simulink model "Vereinfachte_Drehtellersteuerung"  (R2021b)
settings: Solver=ode3  StartTime=0.0  StopTime=10.0  FixedStep=0.01  RelTol=1e-3
values from neighbouring files (symbols this model uses):
  A = 5    [Parametriesierung.m]
  I = 0.5    [Parametriesierung.m]
  igetr = 1080    [Parametriesierung.m]
  K = 8    [Parametriesierung.m]
  MRK = 1    [Parametriesierung.m]
  PHI = 0.001    [Parametriesierung.m]
  Ra = 40    [Parametriesierung.m]
  U = 24    [Parametriesierung.m]
settings Model: Creator=mwjae  LastModifiedBy=mwjae

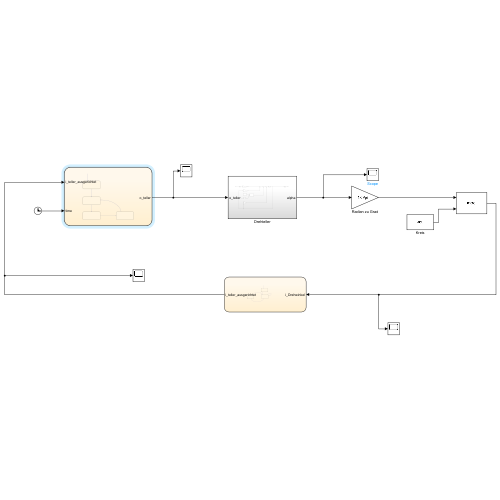
[thumbnail: Simulink's stored preview of the top-level diagram]
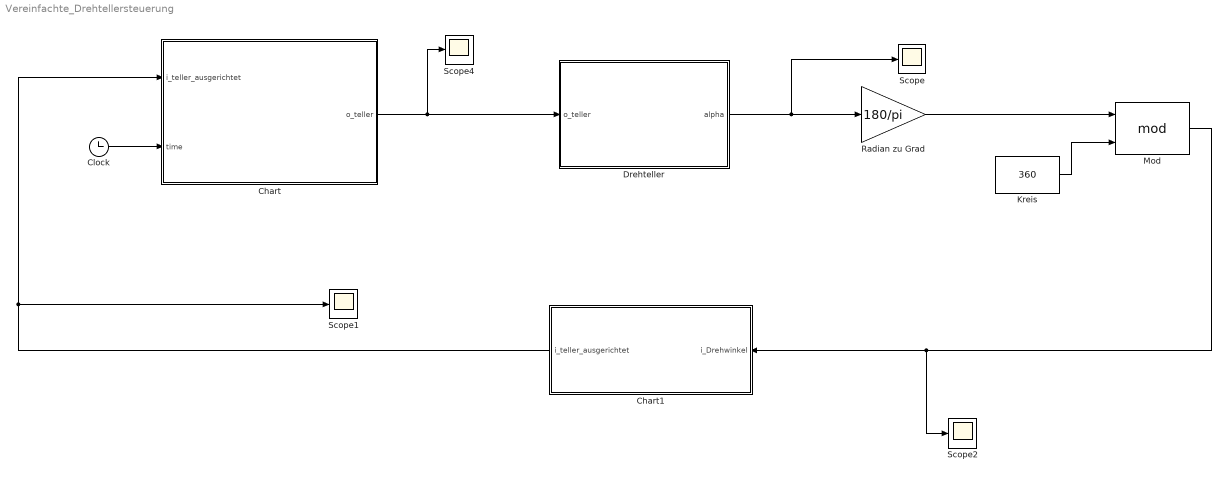
== system Vereinfachte_Drehtellersteuerung ==
  Chart : Stateflow chart  TreatAsAtomicUnit=on
  Chart1 : Stateflow chart  TreatAsAtomicUnit=on
  Clock : Clock
  Drehteller : Subsystem
  Kreis : Constant  Value=360
  Mod : Math  Operator=mod  SaturateOnIntegerOverflow=on
  Radian zu Grad : Gain  Gain=180/pi
  Scope{,1..2,4} (4 alike) : Scope
  wires:
  Drehteller/1(alpha) -> Scope/1, Radian zu Grad/1
  Radian zu Grad/1 -> Mod/1
  Kreis/1 -> Mod/2
  Mod/1 -> Scope2/1, Chart1/1(i_Drehwinkel)
  Chart/1(o_teller) -> Scope4/1, Drehteller/1(o_teller)
  Clock/1 -> Chart/2(time)
  Chart1/1(i_teller_ausgerichtet) -> Chart/1(i_teller_ausgerichtet), Scope1/1

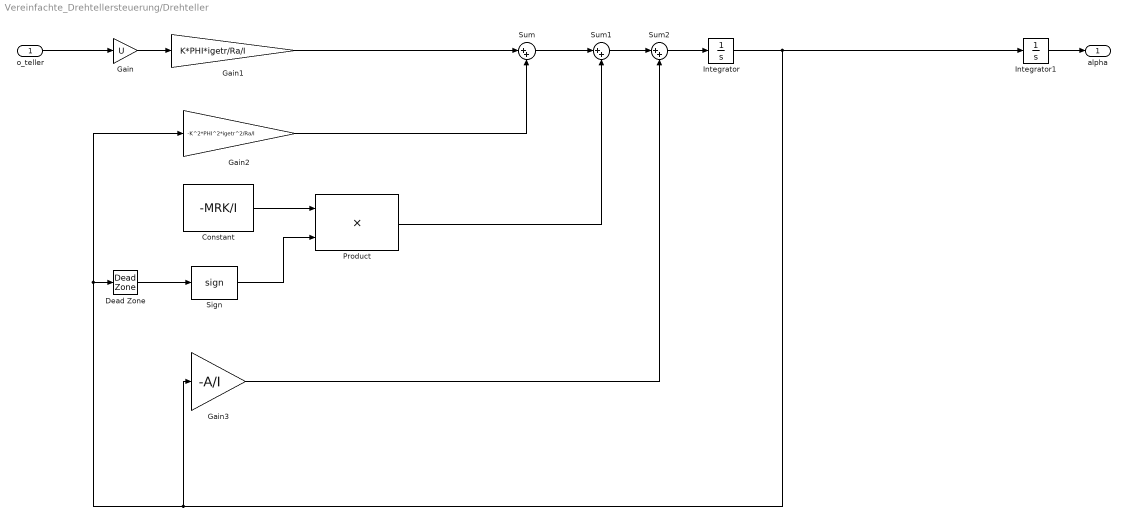
== system Vereinfachte_Drehtellersteuerung/Drehteller ==
  o_teller : Inport
  Constant : Constant  Value=-MRK/I
  Dead Zone : DeadZone  SaturateOnIntegerOverflow=on
  Gain : Gain  Gain=U
  Gain1 : Gain  Gain=K*PHI*igetr/Ra/I
  Gain2 : Gain  Gain=-K^2*PHI^2*igetr^2/Ra/I
  Gain3 : Gain  Gain=-A/I
  Integrator : Integrator
  Integrator1 : Integrator
  Product : Product
  Sign : Signum
  Sum : Sum  Inputs=|++
  Sum1 : Sum  Inputs=|++
  Sum2 : Sum  Inputs=|++
  alpha : Outport
  wires:
  o_teller/1 -> Gain/1
  Gain/1 -> Gain1/1
  Constant/1 -> Product/1
  Sign/1 -> Product/2
  Dead Zone/1 -> Sign/1
  Gain3/1 -> Sum2/2
  Product/1 -> Sum1/2
  Gain1/1 -> Sum/1
  Gain2/1 -> Sum/2
  Sum/1 -> Sum1/1
  Sum1/1 -> Sum2/1
  Sum2/1 -> Integrator/1
  Integrator/1 -> Gain3/1, Gain2/1, Dead Zone/1, Integrator1/1
  Integrator1/1 -> alpha/1

== stateflow chart Vereinfachte_Drehtellersteuerung/Chart1 ==
  state start
  state Ausgerichtet
    i_teller_ausgerichtet = 1;
  state nichtAusgerichtet
    i_teller_ausgerichtet = 0;
  (default) -> start
  start -> Ausgerichtet : [i_Drehwinkel>=88]
  nichtAusgerichtet -> Ausgerichtet : [(0<=mod(i_Drehwinkel,90)&mod(i_Drehwinkel,90)<=2)|(88<=mod(i_Drehwinkel,90)&mod(i_Drehwinkel,90)<90)]
  Ausgerichtet -> Ausgerichtet [order 1] : [(0<=mod(i_Drehwinkel,90)&mod(i_Drehwinkel,90)<=2)|(88<=mod(i_Drehwinkel,90)&mod(i_Drehwinkel,90)<90)]
  Ausgerichtet -> nichtAusgerichtet [order 2] : [(mod(i_Drehwinkel,90)>2 & (mod(i_Drehwinkel,90)<88)|89<mod(i_Drehwinkel,90))]
  data: i_Drehwinkel input; i_teller_ausgerichtet output

== stateflow chart Vereinfachte_Drehtellersteuerung/Chart ==
  state Anfangszustand
    o_teller = 0;
  state Wartenzustand
    o_teller = 0;
  state Drehzustand
    o_teller = 1;
  state Warten_i_teller_ausgerichtet
  (default) -> Anfangszustand
  Anfangszustand -> Wartenzustand
  Warten_i_teller_ausgerichtet -> Wartenzustand : [i_teller_ausgerichtet == 1]
  Wartenzustand -> Drehzustand : after(2,sec)
  Drehzustand -> Warten_i_teller_ausgerichtet : after(0.5,sec)
  data: i_teller_ausgerichtet input; time input; o_teller output
